simulink model "simuMotorFeedforward1"  (R2014a)
settings: Solver=ode45  StartTime=0.0  StopTime=3  MaxStep=0.0001  RelTol=1e-3
values from neighbouring files (symbols this model uses):
  contr = param    [parametres.m]
undefined symbols (not defined in the file or in its folder): param
settings Model: Creator=Etienne  LastModifiedBy=Etienne

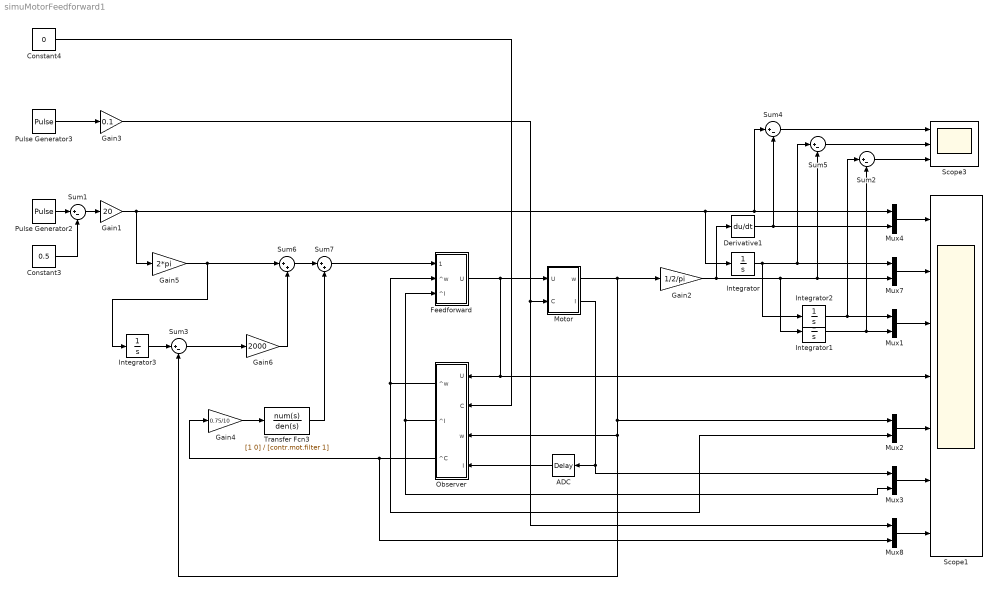
== system simuMotorFeedforward1 ==
  ADC : TransportDelay  DelayTime=param.adc.retard
  Constant3 : Constant  Value=0.5
  Constant4 : Constant  Value=0
  Derivative1 : Derivative
  Feedforward : Subsystem
  Gain1 : Gain  Gain=20
  Gain2 : Gain  Gain=1/2/pi
  Gain3 : Gain  Gain=0.1
  Gain4 : Gain  Gain=0.75/10
  Gain5 : Gain  Gain=2*pi
  Gain6 : Gain  Gain=2000
  Integrator{,1..3} (4 alike) : Integrator
  Motor : Subsystem
  Mux{1..4,7..8} (6 alike) : Mux  Inputs=2
  Observer : Subsystem
  Pulse Generator2 : DiscretePulseGenerator  PulseType=Time based  Period=1  PulseWidth=50  PhaseDelay=0.25/2
  Pulse Generator3 : DiscretePulseGenerator  PulseType=Time based  Period=0.35  PulseWidth=50  PhaseDelay=0.3
  Scope1 : Scope  NumInputPorts=7
      settings: TimeRange=3  YMin=-20~-2~-2~-10~-10~-1~-0.2  YMax=20~4~4~20~30~2~0.2  SaveName=ScopeData2  MaxDataPoints=500000
  Scope3 : Scope  NumInputPorts=3
      settings: TimeRange=3  YMin=-20~-0.004~-9.999999999999999e-06  YMax=20~0.004~5e-05  SaveName=ScopeData3  MaxDataPoints=500000
  Sum{1..5} (5 alike) : Sum  Inputs=|+-
  Sum6 : Sum  Inputs=|++
  Sum7 : Sum  Inputs=|++
  Transfer Fcn3 : TransferFcn  Numerator=[1 0]  Denominator=[contr.mot.filter 1]
  wires:
  Pulse Generator3/1 -> Gain3/1
  Motor/1(w) -> Gain2/1, Observer/3(w), Sum3/2, Mux2/1
  Motor/2(I) -> Mux3/1, ADC/1
  Pulse Generator2/1 -> Sum1/1
  Sum1/1 -> Gain1/1
  Constant3/1 -> Sum1/2
  Gain2/1 -> Mux7/2, Sum5/2, Integrator1/1, Derivative1/1
  Feedforward/1(U) -> Scope1/4, Observer/1(U), Motor/1(U)
  ADC/1 -> Observer/4(I)
  Mux4/1 -> Scope1/1
  Observer/1(^w) -> Feedforward/2(^w), Mux2/2
  Observer/2(^I) -> Feedforward/3(^I), Mux3/2
  Observer/3(^C) -> Gain4/1, Mux8/2
  Gain1/1 -> Mux4/1, Sum4/1, Integrator/1, Gain5/1
  Gain3/1 -> Mux8/1, Motor/2(C)
  Derivative1/1 -> Mux4/2, Sum4/2
  Mux7/1 -> Scope1/2
  Integrator/1 -> Mux7/1, Sum5/1, Integrator2/1
  Mux2/1 -> Scope1/5
  Mux3/1 -> Scope1/6
  Mux8/1 -> Scope1/7
  Sum4/1 -> Scope3/1
  Sum5/1 -> Scope3/2
  Sum7/1 -> Feedforward/1(cons)
  Sum6/1 -> Sum7/1
  Gain5/1 -> Integrator3/1, Sum6/1
  Gain4/1 -> Transfer Fcn3/1
  Mux1/1 -> Scope1/3
  Integrator1/1 -> Sum2/2, Mux1/2
  Integrator2/1 -> Sum2/1, Mux1/1
  Sum2/1 -> Scope3/3
  Integrator3/1 -> Sum3/1
  Sum3/1 -> Gain6/1
  Gain6/1 -> Sum6/2
  Transfer Fcn3/1 -> Sum7/2
  Constant4/1 -> Observer/2(C)

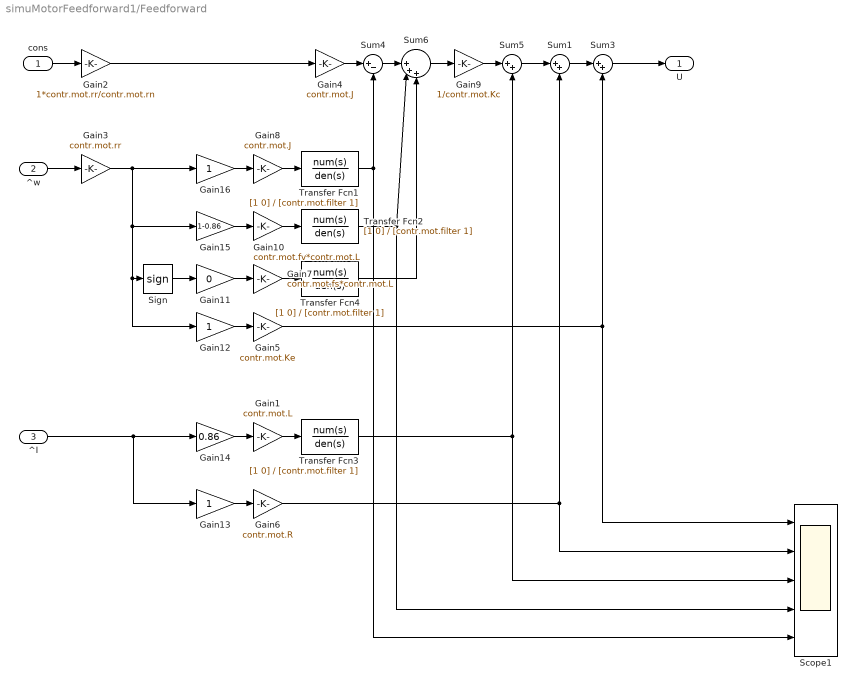
== system simuMotorFeedforward1/Feedforward ==
  cons : Inport
  ^w : Inport  Port=2
  ^I : Inport  Port=3
  Gain1 : Gain  Gain=contr.mot.L
  Gain10 : Gain  Gain=contr.mot.fv*contr.mot.L
  Gain11 : Gain  Gain=0
  Gain12 : Gain
  Gain13 : Gain
  Gain14 : Gain  Gain=0.86
  Gain15 : Gain  Gain=1-0.86
  Gain16 : Gain
  Gain2 : Gain  Gain=1*contr.mot.rr/contr.mot.rn
  Gain3 : Gain  Gain=contr.mot.rr
  Gain4 : Gain  Gain=contr.mot.J
  Gain5 : Gain  Gain=contr.mot.Ke
  Gain6 : Gain  Gain=contr.mot.R
  Gain7 : Gain  Gain=contr.mot.fs*contr.mot.L
  Gain8 : Gain  Gain=contr.mot.J
  Gain9 : Gain  Gain=1/contr.mot.Kc
  Scope1 : Scope  NumInputPorts=5
      settings: TimeRange=3  YMin=-5~-10~-15000~-0.03~-15  YMax=15~10~15000~0.03~15  MaxDataPoints=500000
  Sign : Signum  ZeroCross=off
  Sum1 : Sum  Inputs=|++
  Sum3 : Sum  Inputs=|++
  Sum4 : Sum  Inputs=|+-
  Sum5 : Sum  Inputs=|++
  Sum6 : Sum  Inputs=||+++
  Transfer Fcn{1..4} (4 alike) : TransferFcn  Numerator=[1 0]  Denominator=[contr.mot.filter 1]
  U : Outport
  wires:
  Gain5/1 -> Sum3/2, Scope1/1
  Gain8/1 -> Transfer Fcn1/1
  Gain3/1 -> Gain16/1, Gain15/1, Gain12/1, Sign/1
  Gain2/1 -> Gain4/1
  Sum1/1 -> Sum3/1
  Gain6/1 -> Scope1/2, Sum1/2
  Sum3/1 -> U/1
  Sum6/1 -> Gain9/1
  Transfer Fcn1/1 -> Scope1/5, Sum4/2
  Transfer Fcn3/1 -> Scope1/3, Sum5/2
  Sum5/1 -> Sum1/1
  Gain12/1 -> Gain5/1
  Gain9/1 -> Sum5/1
  Gain1/1 -> Transfer Fcn3/1
  Gain15/1 -> Gain10/1
  Gain16/1 -> Gain8/1
  Gain13/1 -> Gain6/1
  Gain14/1 -> Gain1/1
  Sum4/1 -> Sum6/1
  cons/1 -> Gain2/1
  ^w/1 -> Gain3/1
  ^I/1 -> Gain14/1, Gain13/1
  Gain4/1 -> Sum4/1
  Gain10/1 -> Transfer Fcn2/1
  Transfer Fcn2/1 -> Sum6/2, Scope1/4
  Gain7/1 -> Transfer Fcn4/1
  Gain11/1 -> Gain7/1
  Sign/1 -> Gain11/1
  Transfer Fcn4/1 -> Sum6/3

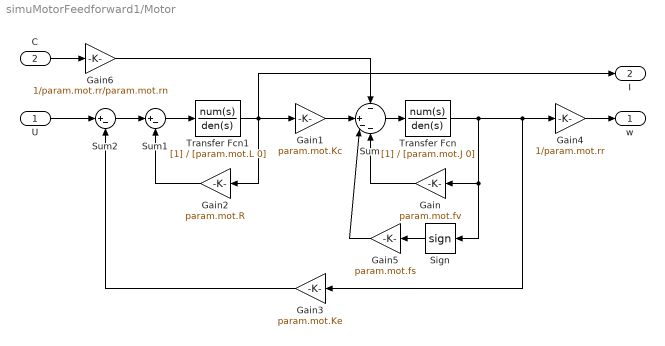
== system simuMotorFeedforward1/Motor ==
  U : Inport
  C : Inport  Port=2
  Gain : Gain  Gain=param.mot.fv
  Gain1 : Gain  Gain=param.mot.Kc
  Gain2 : Gain  Gain=param.mot.R
  Gain3 : Gain  Gain=param.mot.Ke
  Gain4 : Gain  Gain=1/param.mot.rr
  Gain5 : Gain  Gain=param.mot.fs
  Gain6 : Gain  Gain=1/param.mot.rr/param.mot.rn
  Sign : Signum  ZeroCross=off
  Sum : Sum  Inputs=-|+--
  Sum1 : Sum  Inputs=|+-
  Sum2 : Sum  Inputs=|+-
  Transfer Fcn : TransferFcn  Denominator=[param.mot.J 0]
  Transfer Fcn1 : TransferFcn  Denominator=[param.mot.L 0]
  w : Outport
  I : Outport  Port=2
  wires:
  Gain1/1 -> Sum/2
  Transfer Fcn/1 -> Gain3/1, Gain4/1, Sign/1, Gain/1
  Gain3/1 -> Sum2/2
  Sum2/1 -> Sum1/1
  Gain2/1 -> Sum1/2
  Sum1/1 -> Transfer Fcn1/1
  U/1 -> Sum2/1
  C/1 -> Gain6/1
  Gain6/1 -> Sum/1
  Gain4/1 -> w/1
  Sum/1 -> Transfer Fcn/1
  Transfer Fcn1/1 -> Gain1/1, I/1, Gain2/1
  Sign/1 -> Gain5/1
  Gain/1 -> Sum/4
  Gain5/1 -> Sum/3

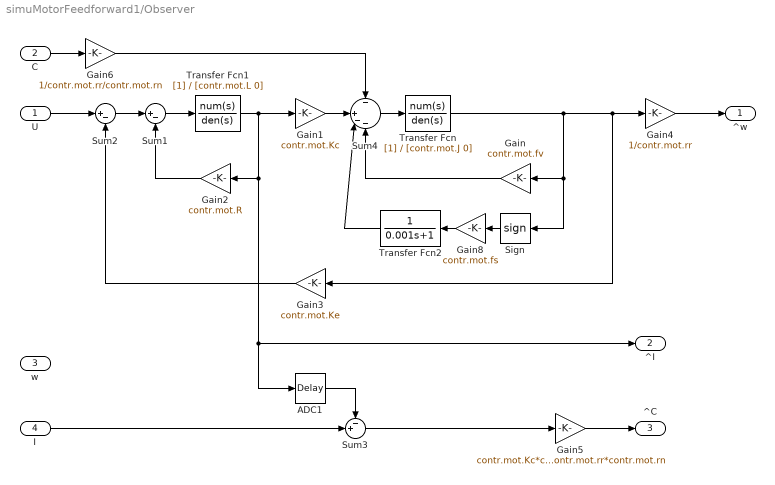
== system simuMotorFeedforward1/Observer ==
  U : Inport
  C : Inport  Port=2
  w : Inport  Port=3
  I : Inport  Port=4
  ADC1 : TransportDelay  DelayTime=contr.adc.retard
  Gain : Gain  Gain=contr.mot.fv
  Gain1 : Gain  Gain=contr.mot.Kc
  Gain2 : Gain  Gain=contr.mot.R
  Gain3 : Gain  Gain=contr.mot.Ke
  Gain4 : Gain  Gain=1/contr.mot.rr
  Gain5 : Gain  Gain=contr.mot.Kc*contr.mot.rr*contr.mot.rn
  Gain6 : Gain  Gain=1/contr.mot.rr/contr.mot.rn
  Gain8 : Gain  Gain=contr.mot.fs
  Sign : Signum  ZeroCross=off
  Sum1 : Sum  Inputs=|+-
  Sum2 : Sum  Inputs=|+-
  Sum3 : Sum  Inputs=-+|
  Sum4 : Sum  Inputs=-|+--
  Transfer Fcn : TransferFcn  Denominator=[contr.mot.J 0]
  Transfer Fcn1 : TransferFcn  Denominator=[contr.mot.L 0]
  Transfer Fcn2 : TransferFcn  Denominator=[0.001 1]
  ^w : Outport
  ^I : Outport  Port=2
  ^C : Outport  Port=3
  wires:
  Transfer Fcn/1 -> Gain3/1, Gain4/1, Gain/1, Sign/1
  Gain3/1 -> Sum2/2
  Sum2/1 -> Sum1/1
  Sum1/1 -> Transfer Fcn1/1
  U/1 -> Sum2/1
  C/1 -> Gain6/1
  Transfer Fcn1/1 -> ^I/1, ADC1/1, Gain2/1, Gain1/1
  Sum3/1 -> Gain5/1
  I/1 -> Sum3/2
  Gain5/1 -> ^C/1
  ADC1/1 -> Sum3/1
  Gain2/1 -> Sum1/2
  Gain4/1 -> ^w/1
  Sign/1 -> Gain8/1
  Gain/1 -> Sum4/4
  Sum4/1 -> Transfer Fcn/1
  Gain1/1 -> Sum4/2
  Gain6/1 -> Sum4/1
  Gain8/1 -> Transfer Fcn2/1
  Transfer Fcn2/1 -> Sum4/3
